simulink library "findClosetPt_tgtPt_SlipAngle"  (R2020a)
settings: Solver=VariableStepAuto  StartTime=0.0  StopTime=10.0  RelTol=1e-3
settings Model: Creator=Ayaz  LastModifiedBy=Ayaz

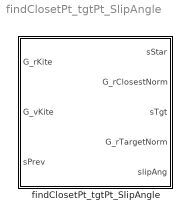
== system findClosetPt_tgtPt_SlipAngle ==
  findClosetPt_tgtPt_SlipAngle : Subsystem  mask{PW=60, PH=28, PE=30, L1=0.05}
      mask prompts: PW "Path width [deg]"; PH "Path height [deg]"; PE "Path mean elevation [deg]"; L1 "Normalized target forward length"
      mask init:
      | aBooth = 0.5*PW*pi/180;
      | bBooth = (1/(2*sqrt(2)))*sqrt(-(PW*pi/180)^2 +sqrt(((PH*pi/180)^2*(4+(PH*pi/180)^2)*(PW*pi/180)^4))/((PH*pi/180)^2));
      | meanEl = PE*pi/180;

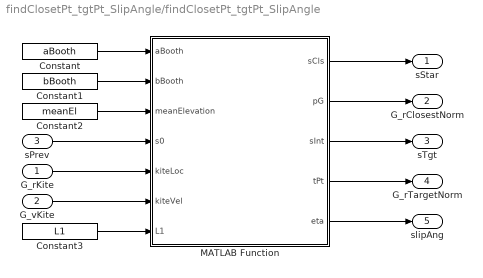
== system findClosetPt_tgtPt_SlipAngle/findClosetPt_tgtPt_SlipAngle ==
  G_rKite : Inport
  G_vKite : Inport  Port=2
  sPrev : Inport  Port=3
  Constant : Constant  Value=aBooth
  Constant1 : Constant  Value=bBooth
  Constant2 : Constant  Value=meanEl
  Constant3 : Constant  Value=L1
  MATLAB Function : MATLAB Function  TreatAsAtomicUnit=on
  sStar : Outport  PortDimensions=1
  G_rClosestNorm : Outport  Port=2  PortDimensions=3
  sTgt : Outport  Port=3  PortDimensions=1
  G_rTargetNorm : Outport  Port=4  PortDimensions=3
  slipAng : Outport  Port=5  PortDimensions=1
  wires:
  G_rKite/1 -> MATLAB Function/5(kiteLoc)
  G_vKite/1 -> MATLAB Function/6(kiteVel)
  sPrev/1 -> MATLAB Function/4(s0)
  MATLAB Function/1(sCls) -> sStar/1
  MATLAB Function/3(sInt) -> sTgt/1
  MATLAB Function/5(eta) -> slipAng/1
  MATLAB Function/2(pG) -> G_rClosestNorm/1
  MATLAB Function/4(tPt) -> G_rTargetNorm/1
  Constant/1 -> MATLAB Function/1(aBooth)
  Constant1/1 -> MATLAB Function/2(bBooth)
  Constant2/1 -> MATLAB Function/3(meanElevation)
  Constant3/1 -> MATLAB Function/7(L1)

== matlab function findClosetPt_tgtPt_SlipAngle/MATLAB Function ==
  data: aBooth input; sCls output; pG output; bBooth input; meanElevation input; s0 input; kiteLoc input; kiteVel input; L1 input; sInt output; tPt output; eta output
function [sCls,pG,sInt,tPt,eta] = findIntersectionPoint(aBooth,bBooth,...
    meanElevation,s0,kiteLoc,kiteVel,L1)

[sCls,pG,sInt,tPt,eta] = findIntersectionPoint(aBooth,bBooth,...
    meanElevation,s0,kiteLoc,kiteVel,L1);

end
